simulink model "test06"  (Simulink 7.4)
settings: Solver=ode3  StartTime=0.0  StopTime=inf  RelTol=1e-3
undefined symbols (not defined in the file or in its folder): serial
libraries: instrumentlib x2
settings Model: Creator=djulzz  LastModifiedBy=djulzz
settings DebuggingCC: SolverPrmCheckMsg=none

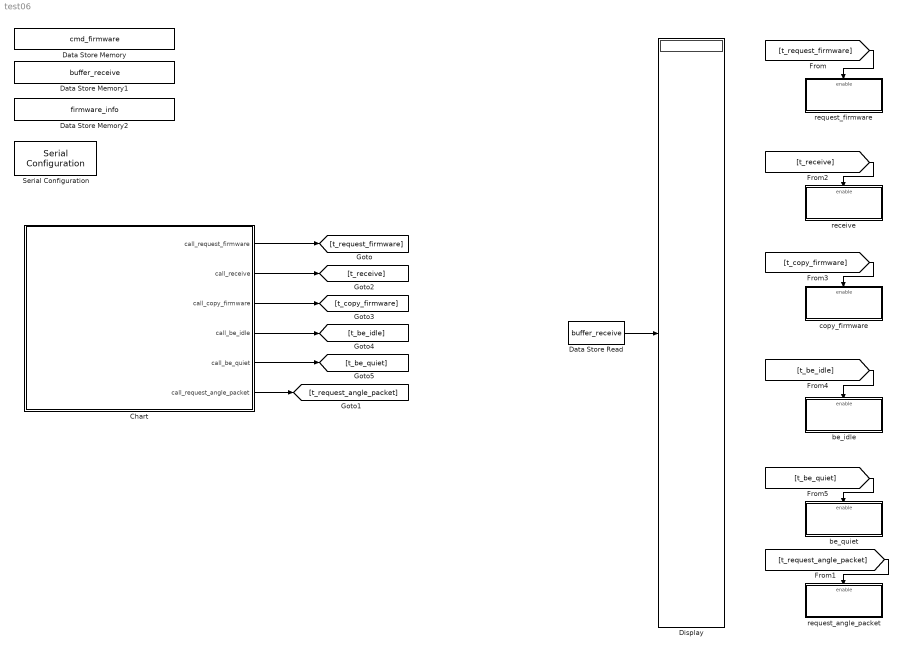
== system test06 ==
  Chart : Stateflow chart
  Data Store Memory : DataStoreMemory  DataStoreName=cmd_firmware  InitialValue=[0 0 0 0 0]  DataType=uint8  OutDataType=fixdt(1, 16)  OutScaling=2^0  OutDataTypeStr=uint8
  Data Store Memory1 : DataStoreMemory  DataStoreName=buffer_receive  InitialValue=[0; 0; 0; 0; 0; 0; 0; 0; 0; 0; 0; 0; 0; 0; 0; 0; 0; 0; 0; 0; 0; 0; 0; 0; 0; 0; 0; 0; 0; 0; 0; 0; 0; 0; 0; 0; 0; 0; 0; 0]  VectorParams1D=off  DataType=uint8  OutDataType=fixdt(1, 16)  OutScaling=2^0  OutDataTypeStr=uint8
  Data Store Memory2 : DataStoreMemory  DataStoreName=firmware_info  InitialValue=[0; 0; 0; 0; 0; 0; 0; 0; 0; 0; 0; 0; 0; 0; 0; 0; 0; 0; 0; 0; 0; 0; 0; 0; 0; 0; 0; 0; 0; 0; 0; 0; 0; 0; 0; 0; 0; 0; 0; 0]  VectorParams1D=off  DataType=uint8  OutDataType=fixdt(1, 16)  OutScaling=2^0  OutDataTypeStr=uint8
  Data Store Read : DataStoreRead  DataStoreName=buffer_receive  SampleTime=-1
  Display : Display
      settings: Format=hex (Stored Integer)
  Serial Configuration : instrumentlib/Serial Configuration  Priority=-200000  DialogController=instrumentcreatedialog  DialogControllerArgs=DataTag0  ComPortMenu=COM1  ComPort=COM1  ObjConstructor=serial('COM1');  BaudRate=38400  DataBits=8  Parity=none  StopBits=1  FlowControl=none  Timeout=10  ByteOrder=LittleEndian
  be_idle : Subsystem  TreatAsAtomicUnit=on
  be_quiet : Subsystem  TreatAsAtomicUnit=on
  copy_firmware : Subsystem  TreatAsAtomicUnit=on
  receive : Subsystem  TreatAsAtomicUnit=on
  request_angle_packet : Subsystem  TreatAsAtomicUnit=on
  request_firmware : Subsystem  TreatAsAtomicUnit=on
  wires:
  [t_request_firmware] -> request_firmware/Enable
  [t_receive] -> receive/Enable
  [t_copy_firmware] -> copy_firmware/Enable
  [t_be_idle] -> be_idle/Enable
  Data Store Read/1 -> Display/1
  [t_be_quiet] -> be_quiet/Enable
  Chart/1(call_request_firmware) -> [t_request_firmware]
  Chart/5(call_be_quiet) -> [t_be_quiet]
  Chart/4(call_be_idle) -> [t_be_idle]
  Chart/3(call_copy_firmware) -> [t_copy_firmware]
  Chart/2(call_receive) -> [t_receive]
  [t_request_angle_packet] -> request_angle_packet/Enable
  Chart/6(call_request_angle_packet) -> [t_request_angle_packet]

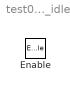
== system test06/be_idle ==
  Enable : EnablePort

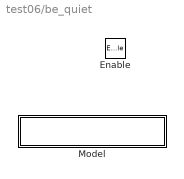
== system test06/be_quiet ==
  Enable : EnablePort
  Model : ModelReference  ModelNameDialog=send_data_rate_model  SimulationMode=Normal  ModelReferenceVersion=1.5  CopyOfModelName=send_data_rate_model

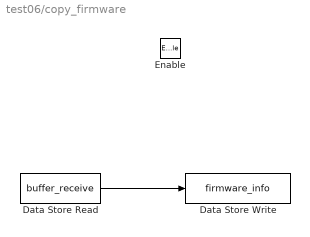
== system test06/copy_firmware ==
  Enable : EnablePort
  Data Store Read : DataStoreRead  DataStoreName=buffer_receive  SampleTime=-1
  Data Store Write : DataStoreWrite  DataStoreName=firmware_info  SampleTime=-1
  wires:
  Data Store Read/1 -> Data Store Write/1

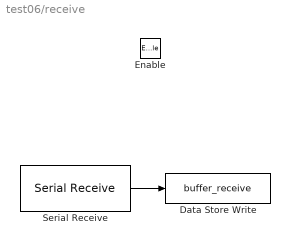
== system test06/receive ==
  Enable : EnablePort
  Data Store Write : DataStoreWrite  DataStoreName=buffer_receive  SampleTime=-1
  Serial Receive : instrumentlib/Serial Receive  DialogController=instrumentcreatedialog  DialogControllerArgs=DataTag1  ComPortMenu=COM1  ComPort=COM1  ObjConstructor=serial('COM1');  Terminator=<none>  DataSize="[40   1]"  DataType=uint8  EnableBlockingMode=on  ActionDataUnavailable=Output last received value  CustomValue=0  SampleTime=-1
  wires:
  Serial Receive/1 -> Data Store Write/1

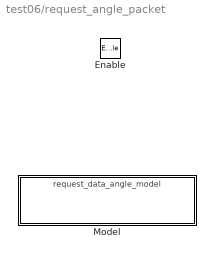
== system test06/request_angle_packet ==
  Enable : EnablePort
  Model : ModelReference  ModelNameDialog=request_data_angle_model  SimulationMode=Normal  ModelReferenceVersion=1.6  CopyOfModelName=request_data_angle_model

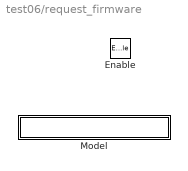
== system test06/request_firmware ==
  Enable : EnablePort
  Model : ModelReference  ModelNameDialog=request_firmware_model  SimulationMode=Normal  ModelReferenceVersion=1.6  CopyOfModelName=request_firmware_model

== stateflow chart Chart ==
  state Step01
    // send the "quiet" command
    call_be_quiet=1;
    call_be_quiet=0;
    call_receive=1;
    call_receive=0;
  state Step02
    // query firmware
    call_request_angle_packet=1;
    call_request_angle_packet=0;
    call_receive=1;
    call_receive=0;
  (default) -> Step01
  Step01 -> Step02
  Step02 -> Step02
  data: cmd_firmware data_store_memory double; buffer_receive data_store_memory double; firmware_info data_store_memory double; call_request_firmware output uint8; call_receive output uint8; call_copy_firmware output uint8; call_be_idle output uint8; call_be_quiet output uint8; call_request_angle_packet output uint8
